simulink model "VB_RI_EKF_GNSS_INS25"  (R2023a)
settings: Solver=FixedStepAuto  StartTime=0  StopTime=200  FixedStep=0.01  RelTol=1e-3
InitFcn:
  | %resilient_initNavigation1216;
  | %init_param;
values from neighbouring files (symbols this model uses):
  C = zeros(n,m)    [utchol.m]
undefined symbols (not defined in the file or in its folder): dt, dtDelay, g0, gam0_rad, GNSSoutragetime, ISUS_flag, magnitude, p, P0, P0_RIEKF, param, pd0, pe0, phi0_rad, pn0, psi, psi0_rad, state_dim, vd0, ve0, vn0
libraries: simulink_extras x133, simulink x81, dspstat3 x81, sharedtransform x69, sharedTrackingLibrary x17, matrix_library x15, deeplib x6, dspfactors x4, aerolibconvert2 x4, aerolibtransform2 x4, dspsrcs4 x1
(part 1 of 32)
settings Model: PacingRate=0.089000  Creator=Ye Xiaoyu  LastModifiedBy=18296
settings DataIOCC: SaveFormat=Structure
settings DebuggingCC: ParameterPrecisionLossMsg=none

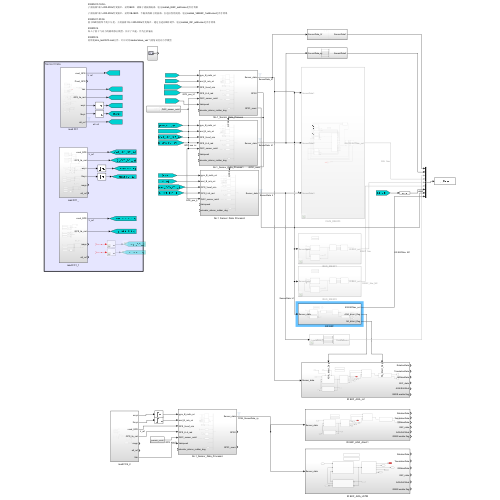
[thumbnail: Simulink's stored preview of the top-level diagram]
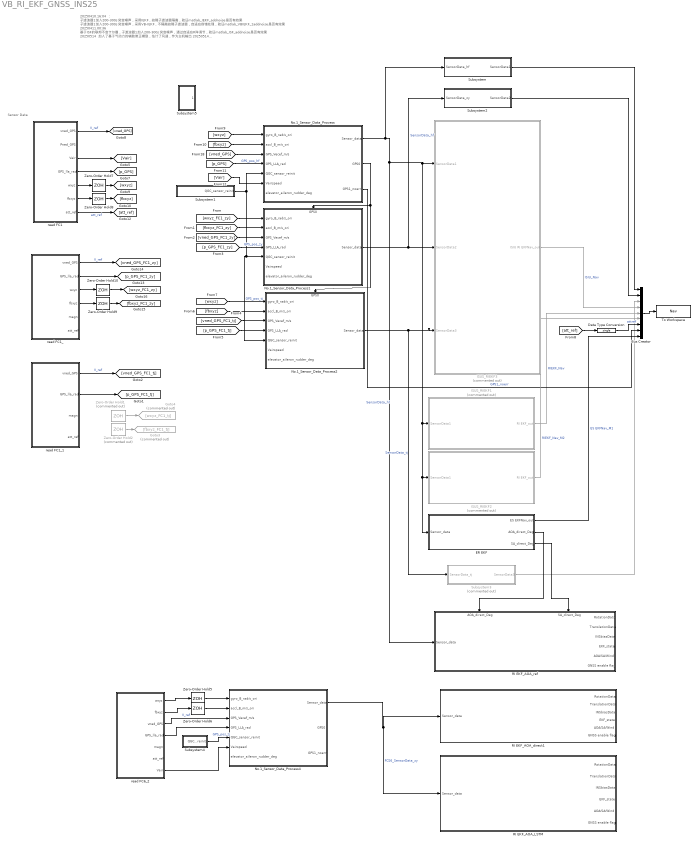
== system VB_RI_EKF_GNSS_INS25 ==
  note: 20250410.16:04：
      | 子滤波器1加入200-300s突变噪声，采用IEKF，故障子滤波器隔离，验证matlab_IEKF_addnoise是否有效果
      |
      | 子滤波器1加入200-300s突变噪声，采用VB-IEKF，不隔离故障子滤波器，自适应容错处理，验证matlab_VBIEKF_1addnoise是否有效果
      |
      | 20250411.00:36
      | 基于ISF的联邦不变卡尔曼，子滤波器1加入200-300s突变噪声，通过自适应R阵调节，验证matlab_ISF_addnoise是否有效果
      |
      | 20250514
      | 加入了基于气动力的辅助修正模型，估计了风速，作为主机输出
      |
      | 20250514
      | 初始化lstm_test0515.mat文件，可以对比master/slave_vair气流角误差动力学模型
  note: Sensor Data
  Bus Creator : BusCreator  Inputs=9
  Data Type Conversion : DataTypeConversion  OutDataTypeStr=single  SaturateOnIntegerOverflow=off  RndMeth=Floor
  ER EKF : Subsystem
  Goto3 : Goto  Commented=on  GotoTag=fbxyz_FC1_tj
  Goto4 : Goto  Commented=on  GotoTag=wxyz_FC1_tj
  ISUS_RIEKF1 : Subsystem  Commented=on
  ISUS_RIEKF2 : Subsystem  Commented=on
  ISUS_RIEKF3 : Subsystem  Commented=on
  No.1_Sensor_Data_Process : Subsystem
  No.1_Sensor_Data_Process1 : Subsystem
      settings: PortSchema="{\"entries\":[{\"content\":{\"sides\":[{\"content\":{\"connectorIds\":[\"In1\",\"In2\",\"In3\",\"In4\",\"In5\",\"In6\",\"In7\"]},\"type\":\"ConnectorPlacement.EquallySpacedRectSide\",\"uuid\":\"9a461442-5a4c-405b-8781-00f946dfe93c\"},{\"content\":{\"connectorIds\":[\"Out1\"],\"side\":\"RIGHT\"},\"type\":\"ConnectorPlacement.EquallySpacedRectSide\",\"uuid\":\"70ca8ff8-5980-4d24-aa39-0c8562a9d1d9\"},{\"content\":{\"connectorIds\":[\"In8\"],\"side\":\"TOP\"},\"type\":\"ConnectorPlacement.EquallySpacedRectSide\",\"uuid\":\"b1ebbd88-9925-4860-b235-fb3cc0770858\"}]},\"type\":\"ConnectorPlacement.EquallySpacedConnector\",\"uuid\":\"3dd6f087-9fad-422a-adf7-c884c798750f\"}],\"packageUris\":[\"http://schema.mathworks.com/mf0/Connector/R2020b\"],\"version\":\"1.0\"}"
  No.1_Sensor_Data_Process2 : Subsystem
      settings: PortSchema="{\"entries\":[{\"content\":{\"sides\":[{\"content\":{\"connectorIds\":[\"In1\",\"In2\",\"In3\",\"In4\",\"In5\",\"In6\",\"In7\"]},\"type\":\"ConnectorPlacement.EquallySpacedRectSide\",\"uuid\":\"9a461442-5a4c-405b-8781-00f946dfe93c\"},{\"content\":{\"connectorIds\":[\"Out1\"],\"side\":\"RIGHT\"},\"type\":\"ConnectorPlacement.EquallySpacedRectSide\",\"uuid\":\"70ca8ff8-5980-4d24-aa39-0c8562a9d1d9\"},{\"content\":{\"connectorIds\":[\"In8\"],\"side\":\"TOP\"},\"type\":\"ConnectorPlacement.EquallySpacedRectSide\",\"uuid\":\"b1ebbd88-9925-4860-b235-fb3cc0770858\"}]},\"type\":\"ConnectorPlacement.EquallySpacedConnector\",\"uuid\":\"3dd6f087-9fad-422a-adf7-c884c798750f\"}],\"packageUris\":[\"http://schema.mathworks.com/mf0/Connector/R2020b\"],\"version\":\"1.0\"}"
  No.1_Sensor_Data_Process4 : Subsystem
  RI EKF_AOA_LSTM : Subsystem
  RI EKF_AOA_direct1 : Subsystem
  RI EKF_AOA_ref : Subsystem
      settings: PortSchema="{\"entries\":[{\"content\":{\"sides\":[{\"content\":{\"connectorIds\":[\"In1\"]},\"type\":\"ConnectorPlacement.EquallySpacedRectSide\",\"uuid\":\"2029a991-91f0-4092-9e34-0b32235deeac\"},{\"content\":{\"connectorIds\":[\"Out1\",\"Out2\",\"Out3\",\"Out4\",\"Out5\",\"Out6\"],\"side\":\"RIGHT\"},\"type\":\"ConnectorPlacement.EquallySpacedRectSide\",\"uuid\":\"c896df0a-2efa-408f-8249-2f9b8aea425e\"},{\"content\":{\"connectorIds\":[\"In2\",\"In3\"],\"side\":\"TOP\"},\"type\":\"ConnectorPlacement.EquallySpacedRectSide\",\"uuid\":\"ea6334ab-d4e0-46e5-a5db-c3c8a7ade9c4\"}]},\"type\":\"ConnectorPlacement.EquallySpacedConnector\",\"uuid\":\"c2bf45d6-b320-4237-b6ce-9fb92476f49c\"}],\"packageUris\":[\"http://schema.mathworks.com/mf0/Connector/R2020b\"],\"version\":\"1.0\"}"
  Subsystem : Subsystem
  Subsystem1 : Subsystem
  Subsystem2 : Subsystem
  Subsystem3 : Subsystem  Commented=on
  Subsystem4 : Subsystem
  Subsystem5 : Subsystem
  To Workspace : ToWorkspace  VariableName=Nav  SaveFormat=Timeseries  SampleTime=0.01
  Zero-Order Hold1 : ZeroOrderHold  Commented=on  SampleTime=dt
  Zero-Order Hold{5..10} (6 alike) : ZeroOrderHold  SampleTime=dt
  Zero-Order Hold2 : ZeroOrderHold  Commented=on  SampleTime=dt
  read FC1 : Subsystem
  read FC1_ : Subsystem
  read FC1_1 : Subsystem
  read FC6_2 : Subsystem
  wires:
  read FC1/1(vned_GPS) -> [vned_GPS]  "V_ref"
  read FC1/6(fbxyz) -> Zero-Order Hold8/1
  read FC1/5(wxyz) -> Zero-Order Hold7/1
  read FC1/7(att_ref) -> [att_ref]  "att_ref"
  read FC1_/2(GPS_lla_rad) -> [p_GPS_FC1_zy]
  read FC1_/1(vned_GPS) -> [vned_GPS_FC1_zy]  "V_ref"
  read FC1/4(GPS_lla_rad) -> [p_GPS]
  Zero-Order Hold10/1 -> [wxyz_FC1_zy]
  Zero-Order Hold9/1 -> [fbxyz_FC1_zy]
  read FC1_/3(wxyz) -> Zero-Order Hold10/1
  read FC1_/4(fbxyz) -> Zero-Order Hold9/1
  Zero-Order Hold7/1 -> [wxyz]
  Zero-Order Hold8/1 -> [fbxyz]
  [fbxyz] -> No.1_Sensor_Data_Process/2(accl_B_m/s_ori)
  Subsystem1/1(QGC_sensor_reinit) -> No.1_Sensor_Data_Process/5(QGC_sensor_reinit), No.1_Sensor_Data_Process1/5(QGC_sensor_reinit), No.1_Sensor_Data_Process2/5(QGC_sensor_reinit)  "GPS_pos_tj"
  [wxyz] -> No.1_Sensor_Data_Process/1(gyro_B_rad/s_ori)
  No.1_Sensor_Data_Process1/1(Sensor_data) -> Subsystem2/1(SensorData_zy), ISUS_RIEKF3/2(SensorData2)  "SensorData_hf"
  [wxyz_FC1_zy] -> No.1_Sensor_Data_Process1/1(gyro_B_rad/s_ori)
  [fbxyz_FC1_zy] -> No.1_Sensor_Data_Process1/2(accl_B_m/s_ori)
  [vned_GPS] -> No.1_Sensor_Data_Process/3(GPS_Vecef_m/s)
  [p_GPS] -> No.1_Sensor_Data_Process/4(GPS_LLA_rad)  "GPS_pos_hf"
  [vned_GPS_FC1_zy] -> No.1_Sensor_Data_Process1/3(GPS_Vecef_m/s)
  [p_GPS_FC1_zy] -> No.1_Sensor_Data_Process1/4(GPS_LLA_rad)  "GPS_pos_zy"
  ? -> Zero-Order Hold2/1
  ? -> Zero-Order Hold1/1
  Zero-Order Hold2/1 -> Goto3/1
  Zero-Order Hold1/1 -> Goto4/1
  read FC1_1/1(vned_GPS) -> [vned_GPS_FC1_tj]  "V_ref"
  read FC1_1/2(GPS_lla_rad) -> [p_GPS_FC1_tj]
  [fbxyz] -> No.1_Sensor_Data_Process2/2(accl_B_m/s_ori)
  [wxyz] -> No.1_Sensor_Data_Process2/1(gyro_B_rad/s_ori)
  [vned_GPS_FC1_tj] -> No.1_Sensor_Data_Process2/3(GPS_Vecef_m/s)
  [p_GPS_FC1_tj] -> No.1_Sensor_Data_Process2/4(GPS_LLA_rad)
  ISUS_RIEKF3/1(ISIU RI EKFNav_out) -> Bus Creator/4  "ISIU_Nav"
  ISUS_RIEKF1/1(RI EKF_out) -> Bus Creator/5  "RIEKF_Nav"
  Bus Creator/1 -> To Workspace/1
  Subsystem/1(SensorData1) -> Bus Creator/1
  Subsystem2/1(SensorData2) -> Bus Creator/2
  Subsystem3/1(SensorData3) -> Bus Creator/3
  [att_ref] -> Data Type Conversion/1
  Data Type Conversion/1 -> Bus Creator/7  "attref"
  No.1_Sensor_Data_Process/2(GPS0) -> No.1_Sensor_Data_Process2/8(GPS0), No.1_Sensor_Data_Process1/8(GPS0)
  No.1_Sensor_Data_Process/3(GPS1_noerr) -> Bus Creator/8  "GPS1_noerr"
  ISUS_RIEKF2/1(RI EKF_out) -> Bus Creator/6  "RIEKF_Nav_M2"
  ER EKF/1(ES EKFNav_out) -> Bus Creator/9  "ES EKFNav_M1"
  No.1_Sensor_Data_Process/1(Sensor_data) -> RI EKF_AOA_ref/1(Sensor_data), ISUS_RIEKF3/1(SensorData1), ISUS_RIEKF2/1(SensorData1), ER EKF/1(Sensor_data), ISUS_RIEKF1/1(SensorData1), Subsystem/1(SensorData_hf)  "SensorData_hf"
  No.1_Sensor_Data_Process2/1(Sensor_data) -> ISUS_RIEKF3/3(SensorData3), Subsystem3/1(SensorData_tj)  "SensorData_tj"
  read FC1/3(Vair) -> [Vair]
  [Vair] -> No.1_Sensor_Data_Process/6(Vairspeed)
  read FC6_2/3(vned_GPS) -> No.1_Sensor_Data_Process4/3(GPS_Vecef_m/s)  "V_ref"
  Zero-Order Hold6/1 -> No.1_Sensor_Data_Process4/2(accl_B_m/s_ori)
  Zero-Order Hold5/1 -> No.1_Sensor_Data_Process4/1(gyro_B_rad/s_ori)
  read FC6_2/2(fbxyz) -> Zero-Order Hold6/1
  read FC6_2/1(wxyz) -> Zero-Order Hold5/1
  Subsystem4/1(QGC_sensor_reinit) -> No.1_Sensor_Data_Process4/5(QGC_sensor_reinit)  "GPS_pos_tj"
  read FC6_2/4(GPS_lla_rad) -> No.1_Sensor_Data_Process4/4(GPS_LLA_rad)
  No.1_Sensor_Data_Process4/1(Sensor_data) -> RI EKF_AOA_LSTM/1(Sensor_data), RI EKF_AOA_direct1/1(Sensor_data)  "FCS6_SensorData_zy"
  read FC6_2/7(Vair) -> No.1_Sensor_Data_Process4/6(Vairspeed)
  ER EKF/2(AOA_direct_Deg) -> RI EKF_AOA_ref/2(AOA_direct_Deg)
  ER EKF/3(SA_direct_Deg) -> RI EKF_AOA_ref/3(SA_direct_Deg)

== system VB_RI_EKF_GNSS_INS25/ER EKF ==
  Sensor_data : Inport
  Bus_Constructor : Subsystem
  Bus_Constructor2 : Subsystem
  Data Store Memory : DataStoreMemory  DataStoreName=feedback_flag_18dim  WriteAfterWriteMsg=warning  ShowAdditionalParam=off
  Data Store Memory1 : DataStoreMemory  DataStoreName=GPS_enable  WriteAfterWriteMsg=warning  ShowAdditionalParam=off
  Data Store Read : DataStoreRead  DataStoreName=GPS_enable  IndexOptions=Index vector (dialog)  Indices=1  OutputSizes=1
  Error State Kalman Filter : Subsystem
  INS propogation : Subsystem
  Scope : Scope
  Scope1 : Scope
  Sensor_data1 : InportShadow
  Subsystem : Subsystem
  ES EKFNav_out : Outport
  AOA_direct_Deg : Outport  Port=2
  SA_direct_Deg : Outport  Port=3
  wires:
  Sensor_data/1 -> INS propogation/1(Sensor_data)
  Error State Kalman Filter/1(delta_state) -> INS propogation/3(delta_state)
  Error State Kalman Filter/2(Measuemrnt Enable Flag) -> INS propogation/2(Measuemrnt Enable Flag)
  INS propogation/1(INSstate) -> Bus_Constructor/1(INSstate), Error State Kalman Filter/2(INS state)
  Sensor_data1/1 -> Error State Kalman Filter/1(Sensor_data)
  Bus_Constructor/1(TranslationData) -> Bus_Constructor2/1(TranlationData)
  Bus_Constructor/2(RotationData) -> Bus_Constructor2/2(RotationData)
  Bus_Constructor/3(INSbiasData) -> Bus_Constructor2/3(INSbiasData)
  Bus_Constructor2/1(RI EKFNav_out) -> Subsystem/1(STD NavData), ES EKFNav_out/1  "RI EKF_out"
  Subsystem/1(AOA_direct_Deg) -> AOA_direct_Deg/1, Scope/1  "AOA_direct_Deg"
  Subsystem/2(SA_direct_Deg) -> SA_direct_Deg/1, Scope1/1  "SA_direct_Deg"

== system VB_RI_EKF_GNSS_INS25/ISUS_RIEKF1 ==
  SensorData1 : Inport
  Bus Selector : BusSelector  OutputSignals=delta_state
  Bus_Constructor : Subsystem
  Bus_Constructor2 : Subsystem
  Data Store Memory : DataStoreMemory  DataStoreName=feedback_flag_18dim_RIEKF  WriteAfterWriteMsg=warning  ShowAdditionalParam=off
  Data Store Memory1 : DataStoreMemory  DataStoreName=GPS_enable_RIEKF  WriteAfterWriteMsg=warning  ShowAdditionalParam=off
  Error State Kalman Filter M1 : Subsystem
  INS propogation : Subsystem
  Sensor_data1 : InportShadow
  RI EKF_out : Outport
  wires:
  Bus_Constructor2/1(RI EKFNav_out) -> RI EKF_out/1  "RI EKF_out"
  Bus_Constructor/4(GNSS enable flag) -> Bus_Constructor2/4(GNSS enable flag)
  Bus_Constructor/3(INSbiasData) -> Bus_Constructor2/3(INSbiasData)  "INSbiasData"
  Bus_Constructor/2(RotationData) -> Bus_Constructor2/2(RotationData)  "RotationData"
  Bus_Constructor/1(TranslationData) -> Bus_Constructor2/1(TranlationData)  "TranslationData"
  Error State Kalman Filter M1/2(EKFstate_M1) -> Bus Selector/1
  SensorData1/1 -> INS propogation/1(Sensor_data)
  Error State Kalman Filter M1/1(Measuemrnt Enable Flag) -> INS propogation/2(Measuemrnt Enable Flag)
  INS propogation/1(INSstate) -> Bus_Constructor/1(INSstate), Error State Kalman Filter M1/2(INS state)
  Sensor_data1/1 -> Error State Kalman Filter M1/1(Sensor_data)
  Bus Selector/1 -> INS propogation/3(delta_state)  "<delta_state>"

== system VB_RI_EKF_GNSS_INS25/ISUS_RIEKF2 ==
  SensorData1 : Inport
  Bus Selector : BusSelector  OutputSignals=delta_state
  Bus_Constructor : Subsystem
  Bus_Constructor2 : Subsystem
  Data Store Memory : DataStoreMemory  DataStoreName=feedback_flag_18dim_RIEKF  WriteAfterWriteMsg=warning  ShowAdditionalParam=off
  Data Store Memory1 : DataStoreMemory  DataStoreName=GPS_enable_RIEKF  WriteAfterWriteMsg=warning  ShowAdditionalParam=off
  Error State Kalman Filter M1 : Subsystem
  INS propogation : Subsystem
  Sensor_data1 : InportShadow
  RI EKF_out : Outport
  wires:
  Bus Selector/1 -> INS propogation/3(delta_state)  "<delta_state>"
  Sensor_data1/1 -> Error State Kalman Filter M1/1(Sensor_data)
  INS propogation/1(INSstate) -> Error State Kalman Filter M1/2(INS state), Bus_Constructor/1(INSstate)
  Error State Kalman Filter M1/1(Measuemrnt Enable Flag) -> INS propogation/2(Measuemrnt Enable Flag)
  SensorData1/1 -> INS propogation/1(Sensor_data)
  Error State Kalman Filter M1/2(EKFstate_M1) -> Bus Selector/1
  Bus_Constructor/1(TranslationData) -> Bus_Constructor2/1(TranlationData)  "TranslationData"
  Bus_Constructor/2(RotationData) -> Bus_Constructor2/2(RotationData)  "RotationData"
  Bus_Constructor/3(INSbiasData) -> Bus_Constructor2/3(INSbiasData)  "INSbiasData"
  Bus_Constructor/4(GNSS enable flag) -> Bus_Constructor2/4(GNSS enable flag)
  Bus_Constructor2/1(RI EKFNav_out) -> RI EKF_out/1  "RI EKF_out"

== system VB_RI_EKF_GNSS_INS25/ISUS_RIEKF3 ==
  SensorData1 : Inport
  SensorData2 : Inport  Port=2
  SensorData3 : Inport  Port=3
  Bus Creator : BusCreator  Inputs=2
  Bus_Constructor : Subsystem
  Bus_Constructor2 : Subsystem
      settings: PortSchema="{\"entries\":[{\"content\":{\"sides\":[{\"content\":{\"connectorIds\":[\"In1\",\"In2\",\"In3\",\"In4\",\"In5\",\"In6\",\"In7\"]},\"type\":\"ConnectorPlacement.EquallySpacedRectSide\",\"uuid\":\"2ada5c99-a5a9-492d-97a7-10d7c05175d7\"},{\"content\":{\"connectorIds\":[\"Out1\"],\"side\":\"RIGHT\"},\"type\":\"ConnectorPlacement.EquallySpacedRectSide\",\"uuid\":\"cde580e4-aba0-41e6-ab1b-1e880cd106da\"},{\"content\":{\"side\":\"TOP\"},\"type\":\"ConnectorPlacement.EquallySpacedRectSide\",\"uuid\":\"542037bf-a2f3-4431-b2f0-0d887f8b5219\"},{\"content\":{\"connectorIds\":[\"In8\"],\"side\":\"BOTTOM\"},\"type\":\"ConnectorPlacement.EquallySpacedRectSide\",\"uuid\":\"59daa5b1-1426-4f22-83e7-df6003f21326\"}]},\"type\":\"ConnectorPlacement.EquallySpacedConnector\",\"uuid\":\"47431650-46c1-4f35-bd73-f1f710c66ac0\"}],\"packageUris\":[\"http://schema.mathworks.com/mf0/Connector/R2020b\"],\"version\":\"1.0\"}"
  Data Store Memory : DataStoreMemory  DataStoreName=feedback_flag_18dim_RIEKF  WriteAfterWriteMsg=warning  ShowAdditionalParam=off
  Data Store Memory1 : DataStoreMemory  DataStoreName=GPS_enable_RIEKF  WriteAfterWriteMsg=warning  ShowAdditionalParam=off
  Error State Kalman Filter M1 : Subsystem
      settings: PortSchema="{\"entries\":[{\"content\":{\"sides\":[{\"content\":{\"connectorIds\":[\"In1\",\"In2\",\"In3\",\"In4\",\"In5\"]},\"type\":\"ConnectorPlacement.EquallySpacedRectSide\",\"uuid\":\"ccab498a-dcb7-4354-abe3-146e031bb9c3\"},{\"content\":{\"connectorIds\":[\"Out1\",\"Out2\",\"Out3\",\"In6\"],\"side\":\"RIGHT\"},\"type\":\"ConnectorPlacement.EquallySpacedRectSide\",\"uuid\":\"6a2d31e3-2b69-4cab-9708-4271f2fce6a7\"},{\"content\":{\"side\":\"TOP\"},\"type\":\"ConnectorPlacement.EquallySpacedRectSide\",\"uuid\":\"b56881dd-3ab1-49f2-a713-f7b000062f7c\"}]},\"type\":\"ConnectorPlacement.EquallySpacedConnector\",\"uuid\":\"3895ce56-28a3-436b-9637-6ade46881fb8\"}],\"packageUris\":[\"http://schema.mathworks.com/mf0/Connector/R2020b\"],\"version\":\"1.0\"}"
  Error State Kalman Filter M2 : Subsystem
  Error State Kalman Filter M3 : Subsystem
  Extract Diagonal1 : matrix_library/Extract Diagonal
  INS propogation : Subsystem
  INS propogation1 : Subsystem
  INS propogation2 : Subsystem
  INS propogation3 : Subsystem
  Reshape : Reshape
  Scope2 : Scope
  Sensor_data1 : InportShadow
  Subsystem : Subsystem
  Terminator : Terminator
  Terminator2 : Terminator
  ISIU RI EKFNav_out : Outport
  wires:
  Extract Diagonal1/1 -> Scope2/1  "covariance_diag"
  Subsystem/1(P_mixed_RIEKF_M1) -> Error State Kalman Filter M1/3(P_mixed_RIEKF_model1)
  Reshape/1 -> Bus Creator/2
  Bus Creator/1 -> Bus_Constructor2/8(ISIU)
  ? -> Reshape/1  "L_k"
  ? -> Bus Creator/1  "mu_k"
  Subsystem/7(X_mixed_RIEKF_M3) -> Error State Kalman Filter M3/4(X_mixed_RIEKF_M3)
  Subsystem/8(P_mixed_RIEKF_M3) -> Error State Kalman Filter M3/3(P_mixed_RIEKF_model3)
  Error State Kalman Filter M3/2(EKFstate_M3) -> Bus_Constructor2/7(EKFstate_M3), Subsystem/3(EKFstate_M3)
  Error State Kalman Filter M3/1(Measuemrnt Enable Flag) -> Terminator2/1
  SensorData3/1 -> Error State Kalman Filter M3/1(Sensor_data)
  Subsystem/6(pk_k) -> Error State Kalman Filter M1/6(pk_k), Extract Diagonal1/1
  Bus_Constructor2/1(RI EKFNav_out) -> ISIU RI EKFNav_out/1  "ISIU RI EKFNav_out"
  Bus_Constructor/4(GNSS enable flag) -> Bus_Constructor2/4(GNSS enable flag)
  Bus_Constructor/3(INSbiasData) -> Bus_Constructor2/3(INSbiasData)  "INSbiasData"
  Bus_Constructor/2(RotationData) -> Bus_Constructor2/2(RotationData)  "RotationData"
  Bus_Constructor/1(TranslationData) -> Bus_Constructor2/1(TranlationData)  "TranslationData"
  Error State Kalman Filter M1/2(EKFstate_M1) -> Bus_Constructor2/5(EKFstate_M1), Subsystem/1(EKFstate_M1)
  Subsystem/4(X_mixed_RIEKF_M2) -> Error State Kalman Filter M2/4(X_mixed_RIEKF_M2)
  Subsystem/3(P_mixed_RIEKF_M2) -> Error State Kalman Filter M2/3(P_mixed_RIEKF_model2)
  Subsystem/2(X_mixed_RIEKF_M1) -> Error State Kalman Filter M1/4(X_mixed_RIEKF_M1)
  Error State Kalman Filter M2/2(EKFstate_M2) -> Bus_Constructor2/6(EKFstate_M2), Subsystem/2(EKFstate_M2)
  Error State Kalman Filter M2/1(Measuemrnt Enable Flag) -> Terminator/1
  SensorData2/1 -> Error State Kalman Filter M2/1(Sensor_data)
  SensorData1/1 -> INS propogation/1(Sensor_data), INS propogation1/1(Sensor_data), INS propogation2/1(Sensor_data), INS propogation3/1(Sensor_data)
  Error State Kalman Filter M1/1(Measuemrnt Enable Flag) -> INS propogation3/2(Measuemrnt Enable Flag), INS propogation2/2(Measuemrnt Enable Flag), INS propogation1/2(Measuemrnt Enable Flag), INS propogation/2(Measuemrnt Enable Flag)
  Sensor_data1/1 -> Error State Kalman Filter M1/1(Sensor_data)
  Error State Kalman Filter M1/3(delta_state) -> INS propogation1/3(delta_state)
  Error State Kalman Filter M3/3(delta_state) -> INS propogation3/3(delta_state)
  Subsystem/5(xk_k) -> INS propogation/3(delta_state)
  INS propogation/1(INSstate) -> Bus_Constructor/1(INSstate)
  Error State Kalman Filter M2/3(delta_state) -> INS propogation2/3(delta_state)
  INS propogation2/1(INSstate) -> Error State Kalman Filter M2/2(INS state)
  INS propogation3/1(INSstate) -> Error State Kalman Filter M3/2(INS state)
  INS propogation1/1(INSstate) -> Error State Kalman Filter M1/2(INS state)
  Subsystem/9(beta_1) -> [beta1]
  [beta1] -> Error State Kalman Filter M1/5(beta-1)
  Subsystem/10(beta_2) -> [beta2]
  Subsystem/11(beta_3) -> [beta3]
  [beta2] -> Error State Kalman Filter M2/5(beta_2)
  [beta3] -> Error State Kalman Filter M3/5(beta_3)

== system VB_RI_EKF_GNSS_INS25/No.1_Sensor_Data_Process ==
  gyro_B_rad/s_ori : Inport
  accl_B_m/s_ori : Inport  Port=2
  GPS_Vecef_m/s : Inport  Port=3
  GPS_LLA_rad : Inport  Port=4
  QGC_sensor_reinit : Inport  Port=5
  Vairspeed : Inport  Port=6
  elevator_aileron_rudder_deg : Inport  Port=7
  Bus Creator : BusCreator  Inputs=8
  Constant3 : Constant
  Constant4 : Constant  Value=0.8
  Data Type Conversion{,1..3,5..6,8..11} (10 alike) : DataTypeConversion  OutDataTypeStr=single  SaturateOnIntegerOverflow=off  RndMeth=Floor
  Data Type Conversion4 : DataTypeConversion  OutDataTypeStr=uint8  SaturateOnIntegerOverflow=off  RndMeth=Floor
  Data Type Conversion7 : DataTypeConversion  OutDataTypeStr=double  SaturateOnIntegerOverflow=off  RndMeth=Floor
  GPS_Data_Process : Subsystem
  IMU_Data_Process : Subsystem
  Magn_Data_Process : Subsystem
  Mux : Mux  Inputs=3
  QGC_sensor_reinit1 : InportShadow  Port=5
  QGC_sensor_reinit2 : InportShadow  Port=5
  Subsystem : Subsystem
  TOF_Data_Process : Subsystem
  baro_Data_Process : Subsystem
  Sensor_data : Outport
  GPS0 : Outport  Port=2
  GPS1_noerr : Outport  Port=3
  wires:
  QGC_sensor_reinit2/1 -> TOF_Data_Process/2(QGC_sensor_reinit)  "QGC_sensor_reinit"
  Data Type Conversion3/1 -> baro_Data_Process/3(baro_tem)
  Data Type Conversion10/1 -> TOF_Data_Process/1(TOF_mm_ori)
  Data Type Conversion6/1 -> Magn_Data_Process/1(magn_B_guass_ori)
  Data Type Conversion5/1 -> baro_Data_Process/1(baro)
  Data Type Conversion9/1 -> GPS_Data_Process/4(hdop_GPS)
  Data Type Conversion4/1 -> GPS_Data_Process/3(GPS_fixtype)
  Data Type Conversion7/1 -> GPS_Data_Process/2(GPS_LLA_rad)
  Data Type Conversion2/1 -> GPS_Data_Process/1(GPS_Vecef_m/s)
  Data Type Conversion1/1 -> IMU_Data_Process/2(accl_B_m/s_ori)
  Data Type Conversion/1 -> IMU_Data_Process/1(gyro_B_rad/s_ori)
  TOF_Data_Process/1(TOF_Data) -> Bus Creator/5
  QGC_sensor_reinit1/1 -> Bus Creator/7  "QGC_sensor_reinit"
  Bus Creator/1 -> Sensor_data/1
  GPS_Vecef_m/s/1 -> Data Type Conversion2/1
  GPS_LLA_rad/1 -> Data Type Conversion7/1
  accl_B_m/s_ori/1 -> Data Type Conversion1/1
  Magn_Data_Process/1(MAGN_Data) -> Bus Creator/4  "MAGN_Data"
  gyro_B_rad/s_ori/1 -> Data Type Conversion/1
  baro_Data_Process/1(BARO_Data) -> Bus Creator/3  "BARO_Data"
  IMU_Data_Process/1(IMU_Data) -> Bus Creator/1  "IMU_Data"
  GPS_Data_Process/1(GPS_Data) -> Bus Creator/2  "GPS_Data"
  QGC_sensor_reinit/1 -> GPS_Data_Process/5(QGC_sensor_reinit), baro_Data_Process/2(QGC_sensor_reinit)  "QGC_sensor_reinit"
  Vairspeed/1 -> Data Type Conversion8/1  "VairspeedData"
  Data Type Conversion8/1 -> Subsystem/1(Vairspeed)
  Subsystem/1(VairspeedData) -> Bus Creator/6
  elevator_aileron_rudder_deg/1 -> Data Type Conversion11/1  "elevator_aileron_rudder_deg"
  Data Type Conversion11/1 -> Bus Creator/8  "elevator_aileron_rudder_deg"
  Constant3/1 -> Data Type Conversion4/1
  Constant4/1 -> Data Type Conversion9/1
  Mux/1 -> Data Type Conversion6/1
  GPS_Data_Process/2(GPS0) -> GPS0/1
  GPS_Data_Process/3(GPS_noerr) -> GPS1_noerr/1

== system VB_RI_EKF_GNSS_INS25/No.1_Sensor_Data_Process1 ==
  gyro_B_rad/s_ori : Inport
  accl_B_m/s_ori : Inport  Port=2
  GPS_Vecef_m/s : Inport  Port=3
  GPS_LLA_rad : Inport  Port=4
  QGC_sensor_reinit : Inport  Port=5
  Vairspeed : Inport  Port=6
  elevator_aileron_rudder_deg : Inport  Port=7
  GPS0 : Inport  Port=8
  Bus Creator : BusCreator  Inputs=8
  Constant3 : Constant
  Constant4 : Constant  Value=0.8
  Data Type Conversion{,1..3,5..6,8..11} (10 alike) : DataTypeConversion  OutDataTypeStr=single  SaturateOnIntegerOverflow=off  RndMeth=Floor
  Data Type Conversion4 : DataTypeConversion  OutDataTypeStr=uint8  SaturateOnIntegerOverflow=off  RndMeth=Floor
  Data Type Conversion7 : DataTypeConversion  OutDataTypeStr=double  SaturateOnIntegerOverflow=off  RndMeth=Floor
  GPS_Data_Process : Subsystem
  IMU_Data_Process : Subsystem
  Magn_Data_Process : Subsystem
  Mux : Mux  Inputs=3
  QGC_sensor_reinit1 : InportShadow  Port=5
  QGC_sensor_reinit2 : InportShadow  Port=5
  Subsystem : Subsystem
  TOF_Data_Process : Subsystem
  baro_Data_Process : Subsystem
  Sensor_data : Outport
  wires:
  Mux/1 -> Data Type Conversion6/1
  Constant4/1 -> Data Type Conversion9/1
  Constant3/1 -> Data Type Conversion4/1
  Data Type Conversion11/1 -> Bus Creator/8  "elevator_aileron_rudder_deg"
  elevator_aileron_rudder_deg/1 -> Data Type Conversion11/1  "elevator_aileron_rudder_deg"
  Subsystem/1(VairspeedData) -> Bus Creator/6
  Data Type Conversion8/1 -> Subsystem/1(Vairspeed)
  Vairspeed/1 -> Data Type Conversion8/1  "VairspeedData"
  QGC_sensor_reinit/1 -> baro_Data_Process/2(QGC_sensor_reinit), GPS_Data_Process/5(QGC_sensor_reinit)  "QGC_sensor_reinit"
  GPS_Data_Process/1(GPS_Data) -> Bus Creator/2  "GPS_Data"
  IMU_Data_Process/1(IMU_Data) -> Bus Creator/1  "IMU_Data"
  baro_Data_Process/1(BARO_Data) -> Bus Creator/3  "BARO_Data"
  gyro_B_rad/s_ori/1 -> Data Type Conversion/1
  Magn_Data_Process/1(MAGN_Data) -> Bus Creator/4  "MAGN_Data"
  accl_B_m/s_ori/1 -> Data Type Conversion1/1
  GPS_LLA_rad/1 -> Data Type Conversion7/1
  GPS_Vecef_m/s/1 -> Data Type Conversion2/1
  Bus Creator/1 -> Sensor_data/1
  QGC_sensor_reinit1/1 -> Bus Creator/7  "QGC_sensor_reinit"
  TOF_Data_Process/1(TOF_Data) -> Bus Creator/5
  Data Type Conversion/1 -> IMU_Data_Process/1(gyro_B_rad/s_ori)
  Data Type Conversion1/1 -> IMU_Data_Process/2(accl_B_m/s_ori)
  Data Type Conversion2/1 -> GPS_Data_Process/1(GPS_Vecef_m/s)
  Data Type Conversion7/1 -> GPS_Data_Process/2(GPS_LLA_rad)
  Data Type Conversion4/1 -> GPS_Data_Process/3(GPS_fixtype)
  Data Type Conversion9/1 -> GPS_Data_Process/4(hdop_GPS)
  Data Type Conversion5/1 -> baro_Data_Process/1(baro)
  Data Type Conversion6/1 -> Magn_Data_Process/1(magn_B_guass_ori)
  Data Type Conversion10/1 -> TOF_Data_Process/1(TOF_mm_ori)
  Data Type Conversion3/1 -> baro_Data_Process/3(baro_tem)
  QGC_sensor_reinit2/1 -> TOF_Data_Process/2(QGC_sensor_reinit)  "QGC_sensor_reinit"
  GPS0/1 -> GPS_Data_Process/6(GPS0)

== system VB_RI_EKF_GNSS_INS25/No.1_Sensor_Data_Process2 ==
  gyro_B_rad/s_ori : Inport
  accl_B_m/s_ori : Inport  Port=2
  GPS_Vecef_m/s : Inport  Port=3
  GPS_LLA_rad : Inport  Port=4
  QGC_sensor_reinit : Inport  Port=5
  Vairspeed : Inport  Port=6
  elevator_aileron_rudder_deg : Inport  Port=7
  GPS0 : Inport  Port=8
  Bus Creator : BusCreator  Inputs=8
  Constant3 : Constant
  Constant4 : Constant  Value=0.8
  Data Type Conversion{,1..3,5..6,8..11} (10 alike) : DataTypeConversion  OutDataTypeStr=single  SaturateOnIntegerOverflow=off  RndMeth=Floor
  Data Type Conversion4 : DataTypeConversion  OutDataTypeStr=uint8  SaturateOnIntegerOverflow=off  RndMeth=Floor
  Data Type Conversion7 : DataTypeConversion  OutDataTypeStr=double  SaturateOnIntegerOverflow=off  RndMeth=Floor
  GPS_Data_Process : Subsystem
  IMU_Data_Process : Subsystem
  Magn_Data_Process : Subsystem
  Mux : Mux  Inputs=3
  QGC_sensor_reinit1 : InportShadow  Port=5
  QGC_sensor_reinit2 : InportShadow  Port=5
  Subsystem : Subsystem
  TOF_Data_Process : Subsystem
  baro_Data_Process : Subsystem
  Sensor_data : Outport
  wires:
  QGC_sensor_reinit2/1 -> TOF_Data_Process/2(QGC_sensor_reinit)  "QGC_sensor_reinit"
  Data Type Conversion3/1 -> baro_Data_Process/3(baro_tem)
  Data Type Conversion10/1 -> TOF_Data_Process/1(TOF_mm_ori)
  Data Type Conversion6/1 -> Magn_Data_Process/1(magn_B_guass_ori)
  Data Type Conversion5/1 -> baro_Data_Process/1(baro)
  Data Type Conversion9/1 -> GPS_Data_Process/4(hdop_GPS)
  Data Type Conversion4/1 -> GPS_Data_Process/3(GPS_fixtype)
  Data Type Conversion7/1 -> GPS_Data_Process/2(GPS_LLA_rad)
  Data Type Conversion2/1 -> GPS_Data_Process/1(GPS_Vecef_m/s)
  Data Type Conversion1/1 -> IMU_Data_Process/2(accl_B_m/s_ori)
  Data Type Conversion/1 -> IMU_Data_Process/1(gyro_B_rad/s_ori)
  TOF_Data_Process/1(TOF_Data) -> Bus Creator/5
  QGC_sensor_reinit1/1 -> Bus Creator/7  "QGC_sensor_reinit"
  Bus Creator/1 -> Sensor_data/1
  GPS_Vecef_m/s/1 -> Data Type Conversion2/1
  GPS_LLA_rad/1 -> Data Type Conversion7/1
  accl_B_m/s_ori/1 -> Data Type Conversion1/1
  Magn_Data_Process/1(MAGN_Data) -> Bus Creator/4  "MAGN_Data"
  gyro_B_rad/s_ori/1 -> Data Type Conversion/1
  baro_Data_Process/1(BARO_Data) -> Bus Creator/3  "BARO_Data"
  IMU_Data_Process/1(IMU_Data) -> Bus Creator/1  "IMU_Data"
  GPS_Data_Process/1(GPS_Data) -> Bus Creator/2  "GPS_Data"
  QGC_sensor_reinit/1 -> GPS_Data_Process/5(QGC_sensor_reinit), baro_Data_Process/2(QGC_sensor_reinit)  "QGC_sensor_reinit"
  Vairspeed/1 -> Data Type Conversion8/1  "VairspeedData"
  Data Type Conversion8/1 -> Subsystem/1(Vairspeed)
  Subsystem/1(VairspeedData) -> Bus Creator/6
  elevator_aileron_rudder_deg/1 -> Data Type Conversion11/1  "elevator_aileron_rudder_deg"
  Data Type Conversion11/1 -> Bus Creator/8  "elevator_aileron_rudder_deg"
  Constant3/1 -> Data Type Conversion4/1
  Constant4/1 -> Data Type Conversion9/1
  Mux/1 -> Data Type Conversion6/1
  GPS0/1 -> GPS_Data_Process/6(GPS0)

== system VB_RI_EKF_GNSS_INS25/No.1_Sensor_Data_Process4 ==
  gyro_B_rad/s_ori : Inport
  accl_B_m/s_ori : Inport  Port=2
  GPS_Vecef_m/s : Inport  Port=3
  GPS_LLA_rad : Inport  Port=4
  QGC_sensor_reinit : Inport  Port=5
  Vairspeed : Inport  Port=6
  elevator_aileron_rudder_deg : Inport  Port=7
  Bus Creator : BusCreator  Inputs=8
  Constant3 : Constant
  Constant4 : Constant  Value=0.8
  Data Type Conversion{,1..3,5..6,8..11} (10 alike) : DataTypeConversion  OutDataTypeStr=single  SaturateOnIntegerOverflow=off  RndMeth=Floor
  Data Type Conversion4 : DataTypeConversion  OutDataTypeStr=uint8  SaturateOnIntegerOverflow=off  RndMeth=Floor
  Data Type Conversion7 : DataTypeConversion  OutDataTypeStr=double  SaturateOnIntegerOverflow=off  RndMeth=Floor
  GPS_Data_Process : Subsystem
  IMU_Data_Process : Subsystem
  Magn_Data_Process : Subsystem
  Mux : Mux  Inputs=3
  QGC_sensor_reinit1 : InportShadow  Port=5
  QGC_sensor_reinit2 : InportShadow  Port=5
  Subsystem : Subsystem
  TOF_Data_Process : Subsystem
  baro_Data_Process : Subsystem
  Sensor_data : Outport
  GPS0 : Outport  Port=2
  GPS1_noerr : Outport  Port=3
  wires:
  GPS_Data_Process/3(GPS_noerr) -> GPS1_noerr/1
  GPS_Data_Process/2(GPS0) -> GPS0/1
  Mux/1 -> Data Type Conversion6/1
  Constant4/1 -> Data Type Conversion9/1
  Constant3/1 -> Data Type Conversion4/1
  Data Type Conversion11/1 -> Bus Creator/8  "elevator_aileron_rudder_deg"
  elevator_aileron_rudder_deg/1 -> Data Type Conversion11/1  "elevator_aileron_rudder_deg"
  Subsystem/1(VairspeedData) -> Bus Creator/6
  Data Type Conversion8/1 -> Subsystem/1(Vairspeed)
  Vairspeed/1 -> Data Type Conversion8/1  "VairspeedData"
  QGC_sensor_reinit/1 -> baro_Data_Process/2(QGC_sensor_reinit), GPS_Data_Process/5(QGC_sensor_reinit)  "QGC_sensor_reinit"
  GPS_Data_Process/1(GPS_Data) -> Bus Creator/2  "GPS_Data"
  IMU_Data_Process/1(IMU_Data) -> Bus Creator/1  "IMU_Data"
  baro_Data_Process/1(BARO_Data) -> Bus Creator/3  "BARO_Data"
  gyro_B_rad/s_ori/1 -> Data Type Conversion/1
  Magn_Data_Process/1(MAGN_Data) -> Bus Creator/4  "MAGN_Data"
  accl_B_m/s_ori/1 -> Data Type Conversion1/1
  GPS_LLA_rad/1 -> Data Type Conversion7/1
  GPS_Vecef_m/s/1 -> Data Type Conversion2/1
  Bus Creator/1 -> Sensor_data/1
  QGC_sensor_reinit1/1 -> Bus Creator/7  "QGC_sensor_reinit"
  TOF_Data_Process/1(TOF_Data) -> Bus Creator/5
  Data Type Conversion/1 -> IMU_Data_Process/1(gyro_B_rad/s_ori)
  Data Type Conversion1/1 -> IMU_Data_Process/2(accl_B_m/s_ori)
  Data Type Conversion2/1 -> GPS_Data_Process/1(GPS_Vecef_m/s)
  Data Type Conversion7/1 -> GPS_Data_Process/2(GPS_LLA_rad)
  Data Type Conversion4/1 -> GPS_Data_Process/3(GPS_fixtype)
  Data Type Conversion9/1 -> GPS_Data_Process/4(hdop_GPS)
  Data Type Conversion5/1 -> baro_Data_Process/1(baro)
  Data Type Conversion6/1 -> Magn_Data_Process/1(magn_B_guass_ori)
  Data Type Conversion10/1 -> TOF_Data_Process/1(TOF_mm_ori)
  Data Type Conversion3/1 -> baro_Data_Process/3(baro_tem)
  QGC_sensor_reinit2/1 -> TOF_Data_Process/2(QGC_sensor_reinit)  "QGC_sensor_reinit"

== system VB_RI_EKF_GNSS_INS25/RI EKF_AOA_LSTM ==
  Sensor_data : Inport
  Bus_Constructor : Subsystem
  Data Store Memory : DataStoreMemory  DataStoreName=feedback_flag_18dim_RIEKF  WriteAfterWriteMsg=warning  ShowAdditionalParam=off
  Data Store Memory1 : DataStoreMemory  DataStoreName=GPS_enable_RIEKF  WriteAfterWriteMsg=warning  ShowAdditionalParam=off
  Error State Kalman Filter : Subsystem
  INS propogation : Subsystem
  Sensor_data1 : InportShadow
  RotationData : Outport
  TranslationData : Outport  Port=2
  INSbiasData : Outport  Port=3
  EKF_state : Outport  Port=4
  AOA/SA/Wind : Outport  Port=5
  GNSS enable flag : Outport  Port=6
  wires:
  Sensor_data1/1 -> Error State Kalman Filter/1(Sensor_data)
  Bus_Constructor/2(RotationData) -> RotationData/1
  Bus_Constructor/1(TranslationData) -> TranslationData/1
  INS propogation/1(INSstate) -> Error State Kalman Filter/2(INS state), Bus_Constructor/1(INSstate)
  Error State Kalman Filter/2(Measuemrnt Enable Flag) -> INS propogation/2(Measuemrnt Enable Flag)
  Error State Kalman Filter/1(delta_state) -> INS propogation/3(delta_state)
  Sensor_data/1 -> INS propogation/1(Sensor_data)
  Error State Kalman Filter/3(EKFstate) -> EKF_state/1
  Bus_Constructor/3(INSbiasData) -> INSbiasData/1
  Bus_Constructor/4(AOA/SA/Wind) -> AOA/SA/Wind/1
  Bus_Constructor/5(GNSS enable flag) -> GNSS enable flag/1

== system VB_RI_EKF_GNSS_INS25/RI EKF_AOA_direct1 ==
  Sensor_data : Inport
  Bus_Constructor : Subsystem
  Bus_Constructor2 : Subsystem
  Data Store Memory : DataStoreMemory  DataStoreName=feedback_flag_18dim_RIEKF  WriteAfterWriteMsg=warning  ShowAdditionalParam=off
  Data Store Memory1 : DataStoreMemory  DataStoreName=GPS_enable_RIEKF  WriteAfterWriteMsg=warning  ShowAdditionalParam=off
  Error State Kalman Filter : Subsystem
  INS propogation : Subsystem
  Scope : Scope
  Scope1 : Scope
  Sensor_data1 : InportShadow
  Subsystem : Subsystem
  RotationData : Outport
  TranslationData : Outport  Port=2
  INSbiasData : Outport  Port=3
  EKF_state : Outport  Port=4
  AOA/SA/Wind : Outport  Port=5
  GNSS enable flag : Outport  Port=6
  wires:
  Bus_Constructor2/1(RI EKFNav_out) -> Subsystem/1(STD NavData)  "RI EKF_out"
  Subsystem/1(AOA_direct_Deg) -> Scope/1  "AOA_direct_Deg"
  Subsystem/2(SA_direct_Deg) -> Scope1/1  "SA_direct_Deg"
  Sensor_data1/1 -> Error State Kalman Filter/1(Sensor_data)
  Bus_Constructor/2(RotationData) -> RotationData/1, Bus_Constructor2/2(RotationData)
  Bus_Constructor/1(TranslationData) -> TranslationData/1, Bus_Constructor2/1(TranlationData)
  INS propogation/1(INSstate) -> Bus_Constructor/1(INSstate), Error State Kalman Filter/2(INS state)
  Error State Kalman Filter/2(Measuemrnt Enable Flag) -> INS propogation/2(Measuemrnt Enable Flag)
  Error State Kalman Filter/1(delta_state) -> INS propogation/3(delta_state)
  Sensor_data/1 -> INS propogation/1(Sensor_data)
  Error State Kalman Filter/3(EKFstate) -> EKF_state/1
  Bus_Constructor/3(INSbiasData) -> INSbiasData/1, Bus_Constructor2/3(INSbiasData)
  Bus_Constructor/4(AOA/SA/Wind) -> AOA/SA/Wind/1
  Bus_Constructor/5(GNSS enable flag) -> GNSS enable flag/1

== system VB_RI_EKF_GNSS_INS25/RI EKF_AOA_ref ==
  Sensor_data : Inport
  AOA_direct_Deg : Inport  Port=2
  SA_direct_Deg : Inport  Port=3
  Bus_Constructor : Subsystem
  Bus_Constructor2 : Subsystem
  Data Store Memory : DataStoreMemory  DataStoreName=feedback_flag_18dim_RIEKF  WriteAfterWriteMsg=warning  ShowAdditionalParam=off
  Data Store Memory1 : DataStoreMemory  DataStoreName=GPS_enable_RIEKF  WriteAfterWriteMsg=warning  ShowAdditionalParam=off
  Error State Kalman Filter : Subsystem
  INS propogation : Subsystem
      settings: PortSchema="{\"entries\":[{\"content\":{\"sides\":[{\"content\":{\"connectorIds\":[\"In1\",\"In2\",\"In3\"]},\"type\":\"ConnectorPlacement.EquallySpacedRectSide\",\"uuid\":\"ad350117-9842-4ab6-bd20-6e86f2cfe10e\"},{\"content\":{\"connectorIds\":[\"Out1\"],\"side\":\"RIGHT\"},\"type\":\"ConnectorPlacement.EquallySpacedRectSide\",\"uuid\":\"ec9cb43b-5599-4786-b87f-a3faeda529a8\"},{\"content\":{\"connectorIds\":[\"In4\",\"In5\"],\"side\":\"TOP\"},\"type\":\"ConnectorPlacement.EquallySpacedRectSide\",\"uuid\":\"5ea40770-eead-4d04-b622-8469fb874ff4\"}]},\"type\":\"ConnectorPlacement.EquallySpacedConnector\",\"uuid\":\"ceab657e-c4bb-4481-b08d-04e739629114\"}],\"packageUris\":[\"http://schema.mathworks.com/mf0/Connector/R2020b\"],\"version\":\"1.0\"}"
  Scope : Scope
  Scope1 : Scope
  Sensor_data1 : InportShadow
  Subsystem : Subsystem
  RotationData : Outport
  TranslationData : Outport  Port=2
  INSbiasData : Outport  Port=3
  EKF_state : Outport  Port=4
  AOA/SA/Wind : Outport  Port=5
  GNSS enable flag : Outport  Port=6
  wires:
  Bus_Constructor/5(GNSS enable flag) -> GNSS enable flag/1
  Bus_Constructor/4(AOA/SA/Wind) -> AOA/SA/Wind/1
  Bus_Constructor/3(INSbiasData) -> Bus_Constructor2/3(INSbiasData), INSbiasData/1
  Error State Kalman Filter/3(EKFstate) -> EKF_state/1
  Sensor_data/1 -> INS propogation/1(Sensor_data)
  Error State Kalman Filter/1(delta_state) -> INS propogation/3(delta_state)
  Error State Kalman Filter/2(Measuemrnt Enable Flag) -> INS propogation/2(Measuemrnt Enable Flag)
  INS propogation/1(INSstate) -> Error State Kalman Filter/2(INS state), Bus_Constructor/1(INSstate)
  Bus_Constructor/1(TranslationData) -> Bus_Constructor2/1(TranlationData), TranslationData/1
  Bus_Constructor/2(RotationData) -> Bus_Constructor2/2(RotationData), RotationData/1
  Sensor_data1/1 -> Error State Kalman Filter/1(Sensor_data)
  Subsystem/2(SA_direct_Deg) -> Scope1/1  "SA_direct_Deg"
  Subsystem/1(AOA_direct_Deg) -> Scope/1  "AOA_direct_Deg"
  Bus_Constructor2/1(RI EKFNav_out) -> Subsystem/1(STD NavData)  "RI EKF_out"
  AOA_direct_Deg/1 -> INS propogation/5(AOA_direct_Deg)
  SA_direct_Deg/1 -> INS propogation/4(SA_direct_Deg)

== system VB_RI_EKF_GNSS_INS25/Subsystem ==
  SensorData_hf : Inport
  Bus Creator1 : BusCreator  Inputs=6
  Bus Selector : BusSelector  OutputSignals=GPS_Data.pos_N_gps,GPS_Data.pos_E_gps,GPS_Data.pos_D_gps,GPS_Data.vn_gps,GPS_Data.ve_gps,GPS_Data.vd_gps
  SensorData1 : Outport
  wires:
  Bus Selector/4 -> Bus Creator1/4  "<vn_gps>"
  Bus Selector/6 -> Bus Creator1/6  "<vd_gps>"
  Bus Selector/1 -> Bus Creator1/1  "<pos_N_gps>"
  SensorData_hf/1 -> Bus Selector/1
  Bus Creator1/1 -> SensorData1/1  "SensorData1"
  Bus Selector/2 -> Bus Creator1/2  "<pos_E_gps>"
  Bus Selector/3 -> Bus Creator1/3  "<pos_D_gps>"
  Bus Selector/5 -> Bus Creator1/5  "<ve_gps>"

== system VB_RI_EKF_GNSS_INS25/Subsystem1 ==
  Compare To Constant : simulink/Logic and Bit Operations/Compare To Constant  relop=<=  const=2.1  OutDataTypeStr=boolean
  Compare To Constant1 : simulink/Logic and Bit Operations/Compare To Constant  relop=>=  const=2  OutDataTypeStr=boolean
  Constant5 : Constant  OutDataTypeStr=uint8
  Constant8 : Constant  Value=0  OutDataTypeStr=uint8
  Digital Clock : DigitalClock  SampleTime=dt
  Logical Operator1 : Logic  AllPortsSameDT=off  OutDataTypeStr=boolean
  Switch3 : Switch  Criteria=u2 > Threshold  SaturateOnIntegerOverflow=off  InputSameDT=off
  QGC_sensor_reinit : Outport
  wires:
  Digital Clock/1 -> Compare To Constant1/1, Compare To Constant/1
  Logical Operator1/1 -> Switch3/2
  Constant5/1 -> Switch3/1
  Compare To Constant1/1 -> Logical Operator1/1
  Compare To Constant/1 -> Logical Operator1/2
  Constant8/1 -> Switch3/3
  Switch3/1 -> QGC_sensor_reinit/1

== system VB_RI_EKF_GNSS_INS25/Subsystem2 ==
  SensorData_zy : Inport
  Bus Creator1 : BusCreator  Inputs=6
  Bus Selector : BusSelector  OutputSignals=GPS_Data.pos_N_gps,GPS_Data.pos_E_gps,GPS_Data.pos_D_gps,GPS_Data.vn_gps,GPS_Data.ve_gps,GPS_Data.vd_gps
  SensorData2 : Outport
  wires:
  Bus Selector/5 -> Bus Creator1/5  "<ve_gps>"
  Bus Selector/3 -> Bus Creator1/3  "<pos_D_gps>"
  Bus Selector/2 -> Bus Creator1/2  "<pos_E_gps>"
  Bus Creator1/1 -> SensorData2/1  "SensorData2"
  SensorData_zy/1 -> Bus Selector/1
  Bus Selector/1 -> Bus Creator1/1  "<pos_N_gps>"
  Bus Selector/6 -> Bus Creator1/6  "<vd_gps>"
  Bus Selector/4 -> Bus Creator1/4  "<vn_gps>"

== system VB_RI_EKF_GNSS_INS25/Subsystem3 ==
  SensorData_tj : Inport
  Bus Creator1 : BusCreator  Inputs=6
  Bus Selector : BusSelector  OutputSignals=GPS_Data.pos_N_gps,GPS_Data.pos_E_gps,GPS_Data.pos_D_gps,GPS_Data.vn_gps,GPS_Data.ve_gps,GPS_Data.vd_gps
  SensorData3 : Outport
  wires:
  Bus Selector/5 -> Bus Creator1/5  "<ve_gps>"
  Bus Selector/3 -> Bus Creator1/3  "<pos_D_gps>"
  Bus Selector/2 -> Bus Creator1/2  "<pos_E_gps>"
  Bus Creator1/1 -> SensorData3/1  "SensorData2"
  SensorData_tj/1 -> Bus Selector/1
  Bus Selector/1 -> Bus Creator1/1  "<pos_N_gps>"
  Bus Selector/6 -> Bus Creator1/6  "<vd_gps>"
  Bus Selector/4 -> Bus Creator1/4  "<vn_gps>"

== system VB_RI_EKF_GNSS_INS25/Subsystem4 ==
  Compare To Constant : simulink/Logic and Bit Operations/Compare To Constant  relop=<=  const=2.1  OutDataTypeStr=boolean
  Compare To Constant1 : simulink/Logic and Bit Operations/Compare To Constant  relop=>=  const=2  OutDataTypeStr=boolean
  Constant5 : Constant  OutDataTypeStr=uint8
  Constant8 : Constant  Value=0  OutDataTypeStr=uint8
  Digital Clock : DigitalClock  SampleTime=dt
  Logical Operator1 : Logic  AllPortsSameDT=off  OutDataTypeStr=boolean
  Switch3 : Switch  Criteria=u2 > Threshold  SaturateOnIntegerOverflow=off  InputSameDT=off
  QGC_sensor_reinit : Outport
  wires:
  Switch3/1 -> QGC_sensor_reinit/1
  Constant8/1 -> Switch3/3
  Compare To Constant/1 -> Logical Operator1/2
  Compare To Constant1/1 -> Logical Operator1/1
  Constant5/1 -> Switch3/1
  Logical Operator1/1 -> Switch3/2
  Digital Clock/1 -> Compare To Constant/1, Compare To Constant1/1

== system VB_RI_EKF_GNSS_INS25/Subsystem5 ==
  Constant18 : Constant  Value=6
  Constant24 : Constant  Value=0.5
  Constant58 : Constant  Value=[5,1,1]
  Constant59 : Constant  Value=3
  Constant60 : Constant  Value=[0,4,0]
  Constant61 : Constant  Value=[0,10,0]
  Constant62 : Constant  Value=0
  Constant63 : Constant  Value=50
  Constant64 : Constant  Value=0
  Constant65 : Constant  Value=pi/3
  Constant66 : Constant  Value=[15,0,0]
  Selector : Selector  InputPortWidth=3  IndexOptions=Index vector (dialog)  Indices=[2]  OutputSizes=1
  Subsystem4 : Subsystem
  V_wind : Outport
  tag scope: T1=global, T2=global, Tc=global, Tg=global, V0=global, Vgmax=global, Vnmax=global, Vrmax=global, Wn=global, distb=global, phiv=global
  wires:
  Constant60/1 -> [V0]
  Constant62/1 -> [T2]
  Constant58/1 -> [Vrmax]
  Constant65/1 -> [Wn]
  Constant59/1 -> [T1]
  Constant66/1 -> [Vgmax]
  Constant64/1 -> [phiv]
  Constant18/1 -> [Tg]
  Constant24/1 -> [distb]
  Constant61/1 -> [Vnmax]
  Constant63/1 -> [Tc]
  Subsystem4/1(V_wind) -> Selector/1
  Selector/1 -> V_wind/1

== system VB_RI_EKF_GNSS_INS25/read FC1 ==
  Add : Sum  Commented=on
  Add1 : Sum
  Bus Creator : BusCreator  Inputs=3
  Bus Creator1 : BusCreator  Inputs=3
  Bus Creator2 : BusCreator  Inputs=3
  Constant : Constant  Commented=on  Value=1.7
  Constant1 : Constant  Value=1.7
  Degrees to Radians : simulink_extras/Transformations/Degrees to Radians
  Degrees to Radians1 : simulink_extras/Transformations/Degrees to Radians
  Degrees to Radians2 : simulink_extras/Transformations/Degrees to Radians
  From Workspace1 : FromWorkspace  VariableName=[time(1:(end-1)),FCS1.data_hf_st.Vn(1:(end-1))]
  From Workspace10 : FromWorkspace  VariableName=[time(1:(end-1)),FCS1.data_hf_st.Ve(1:(end-1))]
  From Workspace11 : FromWorkspace  VariableName=[time(1:(end-1)),FCS1.data_hf_st.Vu(1:(end-1))]
  From Workspace12 : FromWorkspace  VariableName=[time(1:(end-1)),FCS1.data_hf_st.gy(1:(end-1))]
  From Workspace13 : FromWorkspace  VariableName=[time(1:(end-1)),FCS1.data_hf_st.gz(1:(end-1))]
  From Workspace14 : FromWorkspace  VariableName=[time(1:(end-1)),FCS1.data_hf_st.Ax(1:(end-1))]
  From Workspace15 : FromWorkspace  VariableName=[time(1:(end-1)),FCS1.data_hf_st.Ay(1:(end-1))]
  From Workspace16 : FromWorkspace  VariableName=[time(1:(end-1)),FCS1.data_hf_st.Az(1:(end-1))]
  From Workspace17 : FromWorkspace  VariableName=[time(1:(end-1)),FCS1.data_hf_st.roll(1:(end-1))]
  From Workspace18 : FromWorkspace  VariableName=[time(1:(end-1)),FCS1.data_hf_st.pitch(1:(end-1))]
  From Workspace19 : FromWorkspace  VariableName=[time(1:(end-1)),FCS1.data_hf_st.yaw(1:(end-1))]
  From Workspace2 : FromWorkspace  VariableName=[time(1:(end-1)),FCS1.data_hf_st.gx(1:(end-1))]
  From Workspace20 : FromWorkspace  VariableName=[time(1:(end-1)),FCS1.data_hf_st.Vd(1:(end-1))]
  From Workspace3 : FromWorkspace  Commented=on  VariableName=[All.t',All.Yeast]
  From Workspace4 : FromWorkspace  Commented=on  VariableName=[All.t',All.Xnorth]
  From Workspace5 : FromWorkspace  Commented=on  VariableName=[All.t',All.mh]
  From Workspace6 : FromWorkspace  Commented=on  VariableName=[All.t',All.Vc]
  From Workspace7 : FromWorkspace  VariableName=[time(1:(end-1)),FCS1.data_hf_st.lat(1:(end-1))]
  From Workspace8 : FromWorkspace  VariableName=[time(1:(end-1)),FCS1.data_hf_st.lon(1:(end-1))]
  From Workspace9 : FromWorkspace  VariableName=[time(1:(end-1)),FCS1.data_hf_st.height(1:(end-1))]
  Gain : Gain  Commented=on  Gain=1/3.6
  Gain1 : Gain  Gain=-1
  Gain2 : Gain  Commented=on  Gain=-1
  Gain3 : Gain  Gain=1/3.6
  MATLAB Function : MATLAB Function  TreatAsAtomicUnit=on
  Mux : Mux  Inputs=3
  Mux1 : Mux  Inputs=3
  Mux2 : Mux  Inputs=3
  Scope{,1..2,4..10} (10 alike) : Scope
  Scope3 : Scope  Commented=on
  Subsystem : Subsystem
  Subsystem1 : Subsystem
  Subsystem2 : Subsystem
  vned_GPS : Outport
  Pned_GPS : Outport  Port=2
  Vair : Outport  Port=3
  GPS_lla_rad : Outport  Port=4
  wxyz : Outport  Port=5
  fbxyz : Outport  Port=6
  att_ref : Outport  Port=7
  wires:
  Mux/1 -> Scope2/1, vned_GPS/1
  Mux1/1 -> Scope1/1, Pned_GPS/1
  Add/1 -> ?
  Constant/1 -> Add/2
  Degrees to Radians1/1 -> Mux2/2
  Degrees to Radians/1 -> Mux2/1
  From Workspace7/1 -> Degrees to Radians/1  "lat"
  From Workspace8/1 -> Degrees to Radians1/1  "lon"
  Mux2/1 -> GPS_lla_rad/1, Scope/1
  From Workspace9/1 -> Mux2/3  "altitude"
  Gain2/1 -> Mux1/3
  Gain1/1 -> Mux/3
  From Workspace3/1 -> Mux1/2
  From Workspace4/1 -> Mux1/1
  Gain/1 -> Scope3/1, Add/1
  From Workspace6/1 -> Gain/1
  From Workspace1/1 -> Mux/1  "vn"
  From Workspace10/1 -> Mux/2  "ve"
  From Workspace5/1 -> Gain2/1
  From Workspace11/1 -> Gain1/1
  Subsystem/1(y) -> Bus Creator/1
  From Workspace2/1 -> Subsystem/1(u)
  Subsystem1/1(y) -> Bus Creator/2
  From Workspace16/1 -> Bus Creator1/3
  Bus Creator/1 -> Scope4/1, Degrees to Radians2/1
  From Workspace14/1 -> Bus Creator1/1
  From Workspace15/1 -> Bus Creator1/2
  From Workspace12/1 -> Scope7/1, Subsystem1/1(u)
  Degrees to Radians2/1 -> wxyz/1, Scope6/1
  Subsystem2/1(y) -> Bus Creator/3
  From Workspace13/1 -> Subsystem2/1(u)
  Bus Creator1/1 -> fbxyz/1, Scope5/1
  From Workspace19/1 -> MATLAB Function/1(dpsi)
  Bus Creator2/1 -> Scope9/1, att_ref/1, Scope8/1
  From Workspace17/1 -> Bus Creator2/1  "roll"
  From Workspace18/1 -> Bus Creator2/2  "pitch"
  MATLAB Function/1(y) -> Bus Creator2/3  "yaw"
  Gain3/1 -> Add1/1, Scope10/1
  Constant1/1 -> Add1/2
  From Workspace20/1 -> Vair/1, Gain3/1

== system VB_RI_EKF_GNSS_INS25/read FC1_ ==
  Bus Creator : BusCreator  Inputs=3
  Bus Creator1 : BusCreator  Inputs=3
  Bus Creator2 : BusCreator  Inputs=3
  Degrees to Radians : simulink_extras/Transformations/Degrees to Radians
  Degrees to Radians1 : simulink_extras/Transformations/Degrees to Radians
  Degrees to Radians2 : simulink_extras/Transformations/Degrees to Radians
  From Workspace1 : FromWorkspace  VariableName=[time(1:(end-1)),FCS1.data_tj_st.Vn(1:(end-1))]
  From Workspace10 : FromWorkspace  VariableName=[time(1:(end-1)),FCS1.data_tj_st.Ve(1:(end-1))]
  From Workspace11 : FromWorkspace  VariableName=[time(1:(end-1)),FCS1.data_tj_st.Vu(1:(end-1))]
  From Workspace12 : FromWorkspace  VariableName=[time(1:(end-1)),FCS1.data_zy_st.gy(1:(end-1))]
  From Workspace13 : FromWorkspace  VariableName=[time(1:(end-1)),FCS1.data_zy_st.gz(1:(end-1))]
  From Workspace14 : FromWorkspace  VariableName=[time(1:(end-1)),FCS1.data_zy_st.Ax(1:(end-1))]
  From Workspace15 : FromWorkspace  VariableName=[time(1:(end-1)),FCS1.data_zy_st.Ay(1:(end-1))]
  From Workspace16 : FromWorkspace  VariableName=[time(1:(end-1)),FCS1.data_zy_st.Az(1:(end-1))]
  From Workspace17 : FromWorkspace  VariableName=[time(1:(end-1)),FCS1.data_zy_st.roll(1:(end-1))]
  From Workspace18 : FromWorkspace  VariableName=[time(1:(end-1)),FCS1.data_zy_st.pitch(1:(end-1))]
  From Workspace19 : FromWorkspace  VariableName=[time(1:(end-1)),FCS1.data_zy_st.yaw(1:(end-1))]
  From Workspace2 : FromWorkspace  VariableName=[time(1:(end-1)),FCS1.data_zy_st.gx(1:(end-1))]
  From Workspace7 : FromWorkspace  VariableName=[time(1:(end-1)),FCS1.data_zy_st.lat(1:(end-1))]
  From Workspace8 : FromWorkspace  VariableName=[time(1:(end-1)),FCS1.data_zy_st.lon(1:(end-1))]
  From Workspace9 : FromWorkspace  VariableName=[time(1:(end-1)),FCS1.data_zy_st.height(1:(end-1))]
  Gain1 : Gain  Gain=-1
  MATLAB Function : MATLAB Function  TreatAsAtomicUnit=on
  Mux : Mux  Inputs=3
  Mux2 : Mux  Inputs=3
  Mux3 : Mux  Inputs=3
  Scope{,2,4..9} (8 alike) : Scope
  Subsystem : Subsystem
  Subsystem1 : Subsystem
  Subsystem2 : Subsystem
  Zero-Order Hold9 : ZeroOrderHold  SampleTime=dt
  vned_GPS : Outport
  GPS_lla_rad : Outport  Port=2
  wxyz : Outport  Port=3
  fbxyz : Outport  Port=4
  magn : Outport  Port=5
  att_ref : Outport  Port=6
  wires:
  Mux3/1 -> Zero-Order Hold9/1
  From Workspace17/1 -> Bus Creator2/1  "roll"
  From Workspace19/1 -> MATLAB Function/1(dpsi)
  From Workspace11/1 -> Gain1/1
  Bus Creator2/1 -> Scope9/1, att_ref/1, Scope8/1
  Degrees to Radians2/1 -> wxyz/1, Scope6/1
  From Workspace15/1 -> Bus Creator1/2
  Subsystem/1(y) -> Bus Creator/1
  From Workspace14/1 -> Bus Creator1/1
  Zero-Order Hold9/1 -> magn/1
  Degrees to Radians1/1 -> Mux2/2
  Subsystem2/1(y) -> Bus Creator/3
  MATLAB Function/1(y) -> Bus Creator2/3  "yaw"
  From Workspace1/1 -> Mux/1  "vn"
  From Workspace9/1 -> Mux2/3  "altitude"
  Mux/1 -> Scope2/1, vned_GPS/1
  From Workspace16/1 -> Bus Creator1/3
  From Workspace12/1 -> Scope7/1, Subsystem1/1(u)
  From Workspace8/1 -> Degrees to Radians1/1  "lon"
  Bus Creator/1 -> Scope4/1, Degrees to Radians2/1
  Bus Creator1/1 -> fbxyz/1, Scope5/1
  Mux2/1 -> GPS_lla_rad/1, Scope/1
  Gain1/1 -> Mux/3
  From Workspace18/1 -> Bus Creator2/2  "pitch"
  From Workspace10/1 -> Mux/2  "ve"
  Degrees to Radians/1 -> Mux2/1
  Subsystem1/1(y) -> Bus Creator/2
  From Workspace7/1 -> Degrees to Radians/1  "lat"
  From Workspace2/1 -> Subsystem/1(u)
  From Workspace13/1 -> Subsystem2/1(u)
